simulink model "Approximate_id_ad28d30db84132bde97d93811f6c005a2439af74"  (R2020a)
settings: Solver=VariableStepAuto  StartTime=0.0  StopTime=10.0  RelTol=1e-3
model workspace (MAT data in the model file):
  InputValues_20210821T203440345 = [-1 -0.9921875 -0.984375 -0.9765625 -0.96875 -0.9609375 -0.953125 -0.9453125 -0.9375 -0.9296875 -0.921875 -0.9140625 ... (256 elements, 256x1)]
settings Model: Creator=Mahsa  LastModifiedBy=Mahsa

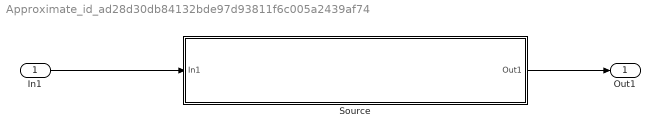
== system Approximate_id_ad28d30db84132bde97d93811f6c005a2439af74 ==
  In1 : Inport  OutDataTypeStr=fixdt(1,8,7)
  Source : Subsystem  Description=This block was created using function approximation.
  Out1 : Outport
  wires:
  In1/1 -> Source/1(In1)
  Source/1(Out1) -> Out1/1

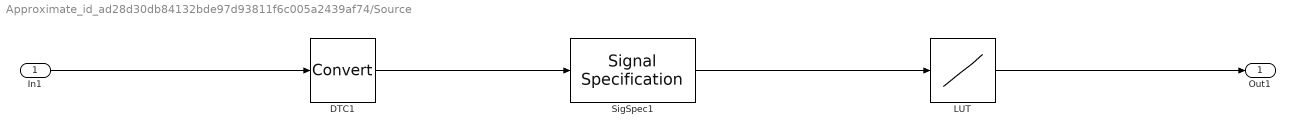
== system Approximate_id_ad28d30db84132bde97d93811f6c005a2439af74/Source ==
  In1 : Inport
  DTC1 : DataTypeConversion  RndMeth=Nearest
  LUT : Lookup_n-D  NumberOfTableDimensions=1  LookupTableObject=FunctionApproximation_LUTObject_20210821T203440330  BreakpointsSpecification=Even spacing  BreakpointsForDimension3=[5, 7]  BreakpointsForDimension1FirstPoint=-1  BreakpointsForDimension1Spacing=0.015625  BreakpointsForDimension1DataTypeStr=numerictype(1,8,7)  IndexSearchMethod=Evenly spaced points  Table=[-0.7578125 -0.7578125 -0.75 -0.7421875 -0.734375 -0.7265625 -0.71875 -0.7109375 -0.703125 -0.6953125 -0.6875 -0.6796875 -0.671875 -0.6640625 -0.65625 -0.640625 -0.6328125 -0.625 -0.6171875 -0.609375 -0.59375 -0.5859375 -0.578125 -0.5625 -0.5546875 -0.546875 -0.53125 -0.5234375 -0.5078125 -0.5 -0.484375 -0.4765625 -0.4609375 -0.453125 -0.4375 -0.421875 -0.4140625 -0.3984375 -0.3828125 -0.375 -0.359375 -0.34375 -0.328125 -0.3203125 -0.3046875 -0.2890625 -0.2734375 -0.2578125 -0.2421875 -0.2265625 -0.21875 -0.203125 -0.1875 -0.171875 -0.15625 -0.140625 -0.125 -0.109375 -0.09375 -0.078125 -0.0625 -0.046875 -0.03125 -0.015625 0 0.015625 0.03125 0.046875 0.0625 0.078125 0.09375 0.109375 0.125 0.140625 0.15625 0.171875 0.1875 0.203125 0.21875 0.2265625 0.2421875 0.2578125 0.2734375 0.2890625 0.3046875 0.3203125 0.328125 0.34375 0.359375 0.375 0.3828125 0.3984375 0.4140625 0.421875 0.4375 0.453125 0.4609375 0.4765625 0.484375 0.5 0.5078125 0.5234375 0.53125 0.546875 0.5546875 0.5625 0.578125 0.5859375 0.59375 0.609375 0.6171875 0.625 0.6328125 0.640625 0.65625 0.6640625 0.671875 0.6796875 0.6875 0.6953125 0.703125 0.7109375 0.71875 0.7265625 0.734375 0.7421875 0.75 0.7578125]  TableDataTypeStr=numerictype(1,8,7)  ExtrapMethod=Clip  UseLastTableValue=on  InternalRulePriority=Speed  OutDataTypeStr=numerictype(1,8,7)  RndMeth=Simplest
  SigSpec1 : SignalSpecification  OutMin=-1  OutMax=0.9921875  OutDataTypeStr=numerictype(1,8,7)
  Out1 : Outport
  wires:
  DTC1/1 -> SigSpec1/1
  SigSpec1/1 -> LUT/1
  LUT/1 -> Out1/1
  In1/1 -> DTC1/1
